simulink model "simulator_3"  (R2018a)
settings: Solver=VariableStepAuto  StartTime=0.0  StopTime=500  RelTol=1e-3
settings Model: Creator=Friends  LastModifiedBy=Friends

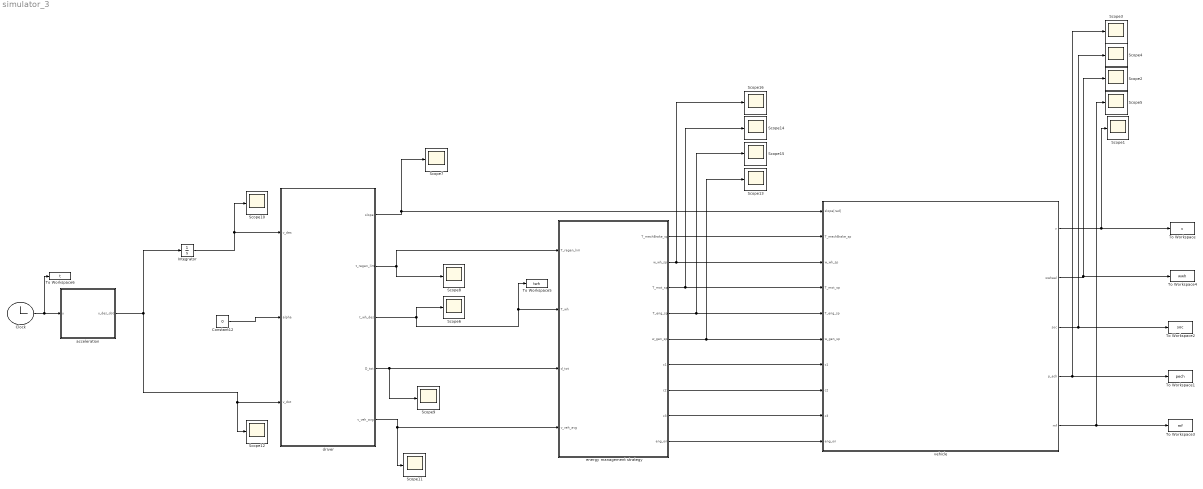
== system simulator_3 ==
  Clock : Clock
  Constant12 : Constant  Value=0
  Integrator : Integrator
  Scope{1..16} (16 alike) : Scope
  To Workspace : ToWorkspace  VariableName=v  SaveFormat=Timeseries  SampleTime=-1
  To Workspace1 : ToWorkspace  VariableName=pech  SaveFormat=Timeseries  SampleTime=-1
  To Workspace2 : ToWorkspace  VariableName=soc  SaveFormat=Timeseries  SampleTime=-1
  To Workspace3 : ToWorkspace  VariableName=mf  SaveFormat=Timeseries  SampleTime=-1
  To Workspace4 : ToWorkspace  VariableName=wwh  SaveFormat=Timeseries  SampleTime=-1
  To Workspace5 : ToWorkspace  VariableName=twh  SaveFormat=Timeseries  SampleTime=-1
  To Workspace6 : ToWorkspace  VariableName=t  SaveFormat=Timeseries  SampleTime=-1
  "acceleration " : MATLAB Function  TreatAsAtomicUnit=on
  driver : MATLAB Function  TreatAsAtomicUnit=on
  "energy management strategy " : MATLAB Function  TreatAsAtomicUnit=on
  vehicle : Subsystem
  wires:
  driver/1(slope) -> Scope7/1, vehicle/1(slope[rad])
  Clock/1 -> To Workspace6/1, "acceleration "/1(u)
  "acceleration "/1(v_des_dot) -> Scope12/1, driver/3(v_dot), Integrator/1
  driver/5(v_veh_avg) -> "energy management strategy "/4(v_veh_avg), Scope11/1
  driver/2(t_regen_lim) -> "energy management strategy "/1(T_regen_lim), Scope8/1
  Integrator/1 -> Scope10/1, driver/1(v_des)
  Constant12/1 -> driver/2(alpha)
  driver/4(D_tot) -> Scope9/1, "energy management strategy "/3(d_tot)
  driver/3(t_wh_des) -> To Workspace5/1, "energy management strategy "/2(T_wh), Scope6/1
  vehicle/1(v) -> Scope1/1, To Workspace/1
  vehicle/2(wwheel) -> To Workspace4/1, Scope2/1
  vehicle/3(soc) -> To Workspace2/1, Scope4/1
  vehicle/4(p_ech) -> To Workspace1/1, Scope3/1
  vehicle/5(mf) -> To Workspace3/1, Scope5/1
  "energy management strategy "/1(T_mechBrake_sp) -> vehicle/2(T_mechBrake_sp)
  "energy management strategy "/2(w_wh_sp) -> Scope16/1, vehicle/3("w_wh_sp ")
  "energy management strategy "/3(T_mot_sp) -> Scope14/1, vehicle/4(T_mot_sp)
  "energy management strategy "/4(T_eng_sp) -> Scope15/1, vehicle/5(T_eng_sp)
  "energy management strategy "/5(w_gen_sp) -> Scope13/1, vehicle/6(w_gen_sp)
  "energy management strategy "/6(c1) -> vehicle/7("c1 ")
  "energy management strategy "/7(c2) -> vehicle/8(c2)
  "energy management strategy "/8(c3) -> vehicle/9(c3)
  "energy management strategy "/9(eng_on) -> vehicle/10(eng_on)

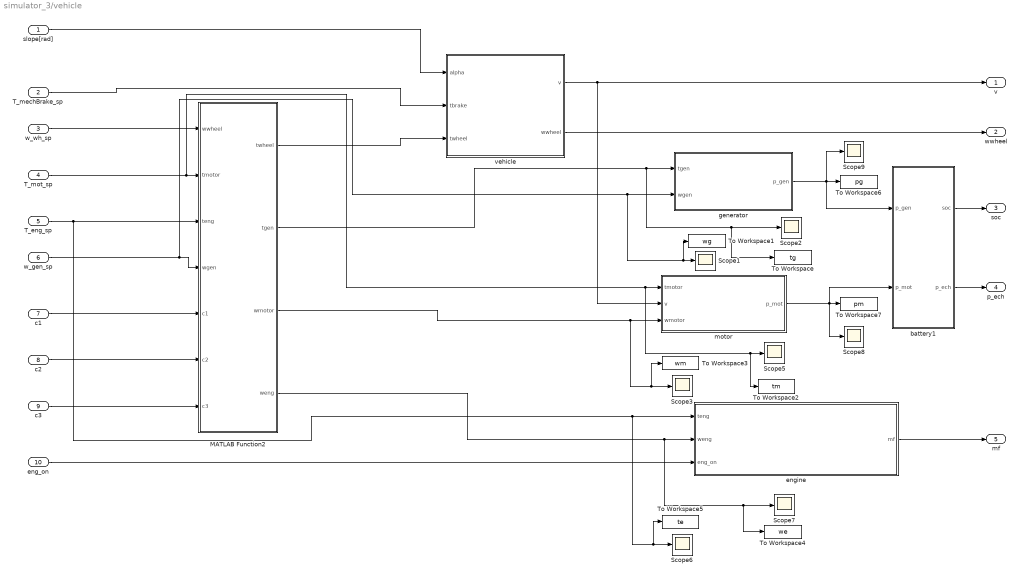
== system simulator_3/vehicle ==
  slope[rad] : Inport
  T_mechBrake_sp : Inport  Port=2
  "w_wh_sp " : Inport  Port=3
  T_mot_sp : Inport  Port=4
  T_eng_sp : Inport  Port=5
  w_gen_sp : Inport  Port=6
  "c1 " : Inport  Port=7
  c2 : Inport  Port=8
  c3 : Inport  Port=9
  eng_on : Inport  Port=10
  MATLAB Function2 : MATLAB Function  TreatAsAtomicUnit=on
  Scope{1..3,5..9} (8 alike) : Scope
  To Workspace : ToWorkspace  VariableName=tg  SaveFormat=Timeseries  SampleTime=-1
  To Workspace1 : ToWorkspace  VariableName=wg  SaveFormat=Timeseries  SampleTime=-1
  To Workspace2 : ToWorkspace  VariableName=tm  SaveFormat=Timeseries  SampleTime=-1
  To Workspace3 : ToWorkspace  VariableName=wm  SaveFormat=Timeseries  SampleTime=-1
  To Workspace4 : ToWorkspace  VariableName=we  SaveFormat=Timeseries  SampleTime=-1
  To Workspace5 : ToWorkspace  VariableName=te  SaveFormat=Timeseries  SampleTime=-1
  To Workspace6 : ToWorkspace  VariableName=pg  SaveFormat=Timeseries  SampleTime=-1
  To Workspace7 : ToWorkspace  VariableName=pm  SaveFormat=Timeseries  SampleTime=-1
  battery1 : Subsystem
  "engine " : Subsystem
  generator : Subsystem
  motor : Subsystem
  vehicle : Subsystem
  v : Outport
  wwheel : Outport  Port=2
  soc : Outport  Port=3
  p_ech : Outport  Port=4
  mf : Outport  Port=5
  wires:
  MATLAB Function2/1(twheel) -> vehicle/3(twheel)
  w_gen_sp/1 -> To Workspace1/1, Scope1/1, generator/2(wgen), MATLAB Function2/4(wgen)
  MATLAB Function2/3(wmotor) -> To Workspace3/1, Scope3/1, motor/3(wmotor)
  vehicle/2(wwheel) -> wwheel/1
  slope[rad]/1 -> vehicle/1(alpha)
  generator/1(p_gen) -> To Workspace6/1, battery1/1(p_gen), Scope9/1
  motor/1(p_mot) -> To Workspace7/1, Scope8/1, battery1/2(p_mot)
  "c1 "/1 -> MATLAB Function2/5(c1)
  MATLAB Function2/4(weng) -> "engine "/2(weng), To Workspace4/1, Scope7/1
  "w_wh_sp "/1 -> MATLAB Function2/1(wwheel)
  vehicle/1(v) -> v/1, motor/2(v)
  c2/1 -> MATLAB Function2/6(c2)
  T_mechBrake_sp/1 -> vehicle/2(tbrake)
  c3/1 -> MATLAB Function2/7(c3)
  T_mot_sp/1 -> To Workspace2/1, Scope5/1, motor/1("tmotor "), MATLAB Function2/2(tmotor)
  T_eng_sp/1 -> "engine "/1(teng), To Workspace5/1, Scope6/1, MATLAB Function2/3(teng)
  battery1/1(soc) -> soc/1
  battery1/2(p_ech) -> p_ech/1
  MATLAB Function2/2(tgen) -> To Workspace/1, Scope2/1, generator/1(tgen)
  eng_on/1 -> "engine "/3(eng_on)
  "engine "/1(mf) -> mf/1

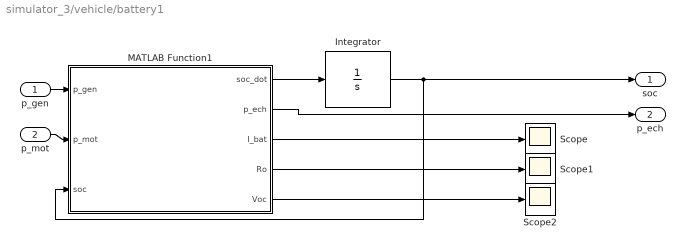
== system simulator_3/vehicle/battery1 ==
  p_gen : Inport
  p_mot : Inport  Port=2
  Integrator : Integrator  InitialCondition=0.95  LimitOutput=on  UpperSaturationLimit=0.95  LowerSaturationLimit=0.3
  MATLAB Function1 : MATLAB Function  TreatAsAtomicUnit=on
  Scope : Scope
  Scope1 : Scope
  Scope2 : Scope
  soc : Outport
  p_ech : Outport  Port=2
  wires:
  MATLAB Function1/1(soc_dot) -> Integrator/1
  Integrator/1 -> MATLAB Function1/3(soc), soc/1
  p_gen/1 -> MATLAB Function1/1(p_gen)
  p_mot/1 -> MATLAB Function1/2(p_mot)
  MATLAB Function1/2(p_ech) -> p_ech/1
  MATLAB Function1/3(I_bat) -> Scope/1
  MATLAB Function1/4(Ro) -> Scope1/1
  MATLAB Function1/5(Voc) -> Scope2/1

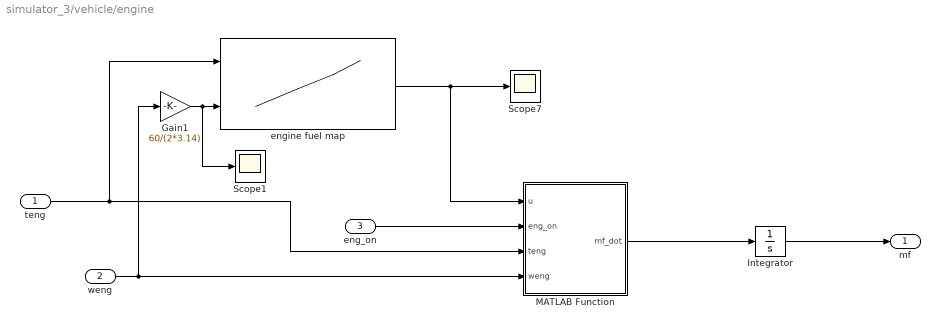
== system simulator_3/vehicle/engine  ==
  teng : Inport
  weng : Inport  Port=2
  eng_on : Inport  Port=3
  Gain1 : Gain  Gain=60/(2*3.14)
  Integrator : Integrator
  MATLAB Function : MATLAB Function  TreatAsAtomicUnit=on
  Scope1 : Scope
  Scope7 : Scope
  engine fuel map : Lookup_n-D  BreakpointsForDimension1=[0,10,20,30,40,50,60,70,80,90,100,110,120,130,140]  BreakpointsForDimension2=[1000,1500,2000,2500,3000,3500,4000,4500,5000]  BreakpointsForDimension3=[5, 7]  Table=reshape([0,0,0,0,0,0,0,0,0,0,0,0,0,0,0,0,0,400,330,300,280,270,260,250,250,250,0,0,0,0,0,0,400,330,300,280,270,260,250,240,240,250,0,0,0,0,0,400,330,300,280,270,250,250,250,240,240,240,0,0,0,0,400,330,300,280,270,250,250,240,240,250,250,0,0,0,0,400,330,300,280,270,260,260,260,260,260,260,260,0,0,0,400,400,300,280,270,270,270,270,270,270,270,270,0,0,0,400,400,400,330,300,300,300,300,300,300,300,300,0,0,0,0,0,0,0,0,0,0,0,0,0,0,0,0],15,9)  DiagnosticForOutOfRangeInput=Warning  InternalRulePriority=Speed  RndMeth=Simplest  InputSameDT=on
  mf : Outport
  wires:
  eng_on/1 -> MATLAB Function/2(eng_on)
  engine fuel map/1 -> Scope7/1, MATLAB Function/1(u)
  Gain1/1 -> Scope1/1, engine fuel map/2
  weng/1 -> MATLAB Function/4(weng), Gain1/1
  teng/1 -> MATLAB Function/3(teng), engine fuel map/1
  MATLAB Function/1(mf_dot) -> Integrator/1
  Integrator/1 -> mf/1

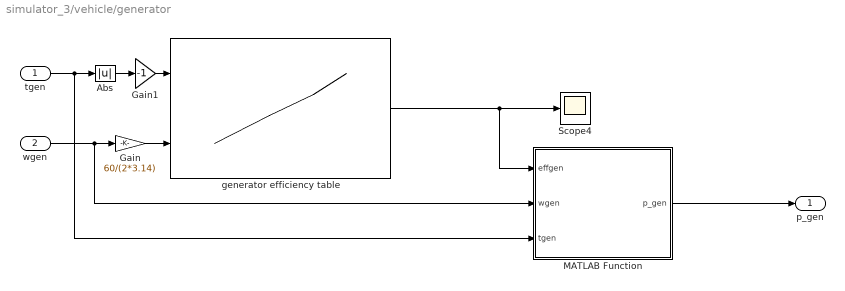
== system simulator_3/vehicle/generator ==
  tgen : Inport
  wgen : Inport  Port=2
  Abs : Abs
  Gain : Gain  Gain=60/(2*3.14)
  Gain1 : Gain  Gain=-1
  MATLAB Function : MATLAB Function  TreatAsAtomicUnit=on
  Scope4 : Scope
  generator efficiency table : Lookup_n-D  BreakpointsForDimension1=[-200,-190,-180,-170,-160,-150,-140,-130,-120,-110,-100,-90,-80,-70,-60,-50,-40,-30,-20,-10,0]  BreakpointsForDimension2=[0,500,1000,1500,2000,2500,3000,3500,4000,4500,5000,5500,6000]  BreakpointsForDimension3=[5, 7]  Table=reshape([0,0,0,0,0,0,0,0,0,0,0,0,0,0,0,0,0,0,0,0,0,0,0,77,77,78,78,79,79,80,80,80,80,81,82,83,84,85,86,87,88,0,0,0,83,83,84,84,85,85,86,86,87,87,88,89,89,90,91,91,91,89,0,0,0,84,85,86,86,87,88,88,89,89,90,90,91,91,92,92,92,92,90,0,0,0,87,88,88,89,89,90,90,90,91,91,92,92,92,93,93,92,92,90,0,0,0,88,89,90,90,91,91,91,91,92,92,92,93,93,93,93,93,92,90,0,0,0,0,90,91,91,92,92,92,92,93,93,93,93,93,94,93,93,92,90,0,0,0,0,91,91,92,92,92,93,93,93,93,93,94,94,94,94,94,93,91,0,0,0,0,0,0,91,92,93,93,93,94,94,94,94,94,94,94,94,93,90,0,0,0,0,0,0,0,0,92,93,93,94,94,94,94,94,94,94,94,93,90,0,0,0,0,0,0,0,0,0,92,92,93,94,94,94,94,94,94,94,93,90,0,0,0,0,0,0,0,0,0,0,92,92,93,94,94,94,94,94,94,93,90,0,0,0,0,0,0,0,0,0,0,0,92,92,93,94,94,94,94,94,93,90,0],21,13)  DiagnosticForOutOfRangeInput=Warning  InternalRulePriority=Speed  RndMeth=Simplest  InputSameDT=on
  p_gen : Outport
  wires:
  generator efficiency table/1 -> Scope4/1, MATLAB Function/1(effgen)
  MATLAB Function/1(p_gen) -> p_gen/1
  tgen/1 -> MATLAB Function/3(tgen), Abs/1
  wgen/1 -> Gain/1, MATLAB Function/2(wgen)
  Gain/1 -> generator efficiency table/2
  Abs/1 -> Gain1/1
  Gain1/1 -> generator efficiency table/1

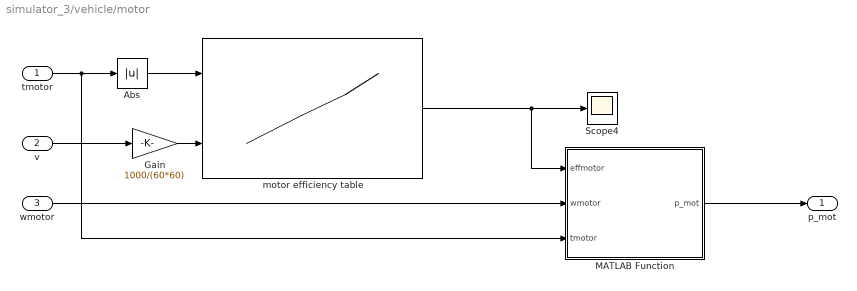
== system simulator_3/vehicle/motor ==
  "tmotor " : Inport
  v : Inport  Port=2
  wmotor : Inport  Port=3
  Abs : Abs
  Gain : Gain  Gain=1000/(60*60)
  MATLAB Function : MATLAB Function  TreatAsAtomicUnit=on
  Scope4 : Scope
  motor efficiency table : Lookup_n-D  BreakpointsForDimension1=[0,250,500,750,1000,1250,1500,1750,2000,2250,2500]  BreakpointsForDimension2=[0,25,50,75,100,125,150,175]  BreakpointsForDimension3=[5, 7]  Table=reshape([69,69,69,69,69,69,69,69,69,69,69,69,70,80,80,80,80,80,80,80,80,80,69,80,84,84,84,84,84,84,84,84,84,69,80,86,88,88,86,86,84,0,0,0,69,80,84,86,86,84,80,0,0,0,0,69,70,80,84,80,0,0,0,0,0,0,69,70,70,70,0,0,0,0,0,0,0,69,70,70,70,0,0,0,0,0,0,0],11,8)  DiagnosticForOutOfRangeInput=Warning  InternalRulePriority=Speed  RndMeth=Simplest  InputSameDT=on
  p_mot : Outport
  wires:
  wmotor/1 -> MATLAB Function/2(wmotor)
  "tmotor "/1 -> MATLAB Function/3(tmotor), Abs/1
  motor efficiency table/1 -> Scope4/1, MATLAB Function/1(effmotor)
  v/1 -> Gain/1
  Gain/1 -> motor efficiency table/2
  MATLAB Function/1(p_mot) -> p_mot/1
  Abs/1 -> motor efficiency table/1

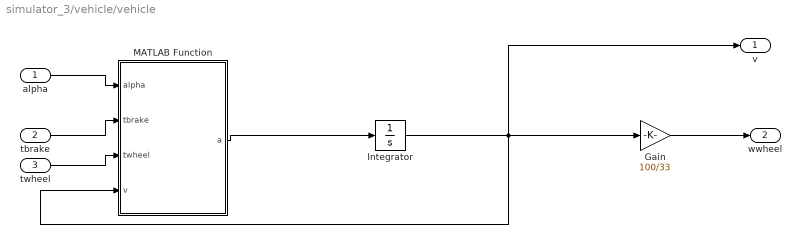
== system simulator_3/vehicle/vehicle ==
  alpha : Inport
  tbrake : Inport  Port=2
  twheel : Inport  Port=3
  Gain : Gain  Gain=100/33
  Integrator : Integrator
  MATLAB Function : MATLAB Function  TreatAsAtomicUnit=on
  v : Outport
  wwheel : Outport  Port=2
  wires:
  Integrator/1 -> MATLAB Function/4(v), Gain/1, v/1
  twheel/1 -> MATLAB Function/3(twheel)
  MATLAB Function/1(a) -> Integrator/1
  tbrake/1 -> MATLAB Function/2(tbrake)
  alpha/1 -> MATLAB Function/1(alpha)
  Gain/1 -> wwheel/1

== matlab function simulator_3/vehicle/vehicle/MATLAB Function ==
  data: alpha input; a output; tbrake input; twheel input; v input
function a = v_dot(alpha, tbrake, twheel, v)
    r_wh = 33e-2; %m
    c0 = 105.95; %N
    c1 = 0.01; %Ns/m
    c2 = 0.4340; %Ns^2/m^2
    Jv = 207; %kg m^2
    wb = 2685e-3; %m
    cogh = 550e-3;%m
    g = 9.81; %m/s^2
    mv = 1812; %kg
    
a =(r_wh/Jv)*(tbrake + twheel - mv*r_wh*g*sin(deg2rad(alpha)) - r_wh*(c0 + c1*v + c2*v*v));

== matlab function simulator_3/vehicle/MATLAB Function2 ==
  data: twheel output; tgen output; wwheel input; tmotor input; teng input; wgen input; c1 input; c2 input; c3 input; wmotor output; weng output
function [twheel,tgen,wmotor,weng] = powertrain(wwheel,tmotor,teng,wgen,c1,c2,c3)
rho=2.24; %nring/nsun
Rd=2.16; %differential gear ratio
% torques in Nm, angular speeds in rad/s
if (c1==1)&&(c2==0)&&(c3==0)
    tgen=0;
    twheel=Rd*(rho+1)*tmotor;
    weng=0;
    wmotor=wwheel*Rd*(rho+1);   
elseif (c1==0)&&(c2==1)&&(c3==0)
    tgen=rho*tmotor;
    twheel=Rd*(rho+1)*tmotor;
    weng=0;
    wmotor=wwheel*Rd*(rho+1)-wgen*rho;
elseif (c1==1)&&(c2==0)&&(c3==1)
    tgen=-teng;
    twheel=Rd*(rho+1)*tmotor;
    weng=wgen;
    wmotor=wwheel*Rd*(rho+1);
elseif (c1==0)&&(c2==1)&&(c3==1)
    tgen=rho*tmotor-teng;
    twheel=Rd*(rho+1)*tmotor;
    weng=wgen;
    wmotor=wwheel*Rd*(rho+1)-rho*wgen;
else
    tgen=0;
    twheel=0;
    weng=0;
    wmotor=0;
end

== matlab function simulator_3/driver ==
  data: v_des input; slope output; alpha input; t_regen_lim output; t_wh_des output; D_tot output; v_veh_avg output; v_dot input
function [slope, t_regen_lim, t_wh_des, D_tot, v_veh_avg]  = fcn(v_des,alpha,v_dot)
slope=alpha;
t_regen_lim = 0;
t_wh_des = (207/0.33)*v_dot + 0.33*(105.95 + 0.01*v_des + 0.434*(v_des*v_des));
D_tot=0;
v_veh_avg=v_des;

== matlab function simulator_3/vehicle/generator/MATLAB Function ==
  data: effgen input; p_gen output; wgen input; tgen input
function p_gen = genpower(effgen,wgen,tgen)
if tgen>0
    p_gen = (power(effgen/100,-1))*wgen*tgen;
else
    p_gen = (power(effgen/100,1))*wgen*tgen;
end

== matlab function simulator_3/energy management strategy  ==
  data: T_mechBrake_sp output; w_wh_sp output; T_mot_sp output; T_eng_sp output; w_gen_sp output; c1 output; c2 output; c3 output; T_regen_lim input; T_wh input; eng_on output; d_tot input; v_veh_avg input
function [T_mechBrake_sp, w_wh_sp, T_mot_sp, T_eng_sp, w_gen_sp, c1, c2, c3, eng_on] = ems(T_regen_lim, T_wh, d_tot, v_veh_avg)
rho=2.24; %nring/nsun
Rd=2.16; %differential gear ratio
r_wh = 33e-2; %m
%{
c1=1;
c2=0;
c3=0;
T_mechBrake_sp=0;
w_wh_sp=v_veh_avg/r_wh;
T_mot_sp=T_wh/(Rd*(rho+1));
T_eng_sp=0;
w_gen_sp=0;
eng_on=0;
%}
%{
c1=0;
c2=1;
c3=0;
T_mechBrake_sp=0;
w_wh_sp=v_veh_avg/r_wh;
T_mot_sp=T_wh/(Rd*(rho+1));
T_eng_sp=0;
w_gen_sp=w_wh_sp*Rd;
eng_on=0;
%}
c1=1;
c2=0;
c3=1;
T_mechBrake_sp=0;
w_wh_sp=v_veh_avg/r_wh;
T_mot_sp=T_wh/(Rd*(rho+1));
T_eng_sp=95;
w_gen_sp=250;
eng_on=1;

== matlab function simulator_3/vehicle/motor/MATLAB Function ==
  data: effmotor input; p_mot output; wmotor input; tmotor input
function p_mot = motpower(effmotor,wmotor,tmotor)
if tmotor>0
    p_mot = (power(effmotor/100,-1))*wmotor*tmotor;
else
    p_mot = (power(effmotor/100,-1))*wmotor*tmotor;
end

== matlab function simulator_3/acceleration  ==
  data: u input; v_des_dot output
function v_des_dot = fcn(u)

v_des_dot = 20*0.5*pi*cos(0.5*pi*u/100)/100;

== matlab function simulator_3/vehicle/battery1/MATLAB Function1 ==
  data: p_gen input; soc_dot output; p_mot input; soc input; p_ech output; I_bat output; Ro output; Voc output
function [soc_dot, p_ech, I_bat, Ro, Voc] = soc_dot(p_gen,p_mot,soc)
n_c=1;
Voc = (-0.5911*(soc*soc) + 1.1892*(soc) + 3.242)*96; %volts
Q = 160000; %As
Ro = 32/1000*(-0.3501*(soc*soc*soc)+0.952*(soc*soc)-0.9387*(soc)+2.2806); %ohms
P_bat = p_gen+p_mot;
I_bat = (Voc-sqrt(Voc^2 - 4*P_bat*Ro))/(2*Ro);
p_ech = Voc*I_bat;
soc_dot = -n_c*I_bat/Q;

== matlab function simulator_3/vehicle/engine /MATLAB Function ==
  data: u input; mf_dot output; eng_on input; teng input; weng input
function mf_dot = fcn(u, eng_on, teng, weng)

mf_dot = u*eng_on*teng*weng/(3.6e+6);
